simulink model "swingup_control"  (R2021a)
settings: Solver=VariableStepAuto  StartTime=0.0  StopTime=10  RelTol=1e-3
undefined symbols (not defined in the file): A, alpha, B, beta, bm, bp, C, fs_IMU, g, J1, Jw, Ke, Ken, Kt, Ku, Kw, L, La, Ra, real_acc_height, t_noise, V_nom, w_deriv, wacc_LPF, wd_IMU, wgyro_LPF, wn, x0, x0_sw
libraries: spsFirstOrderFilterLib x4, simulink x3, dsparch4 x1, dspsigops x1
settings Model: Creator=jpss8  LastModifiedBy=jpss8

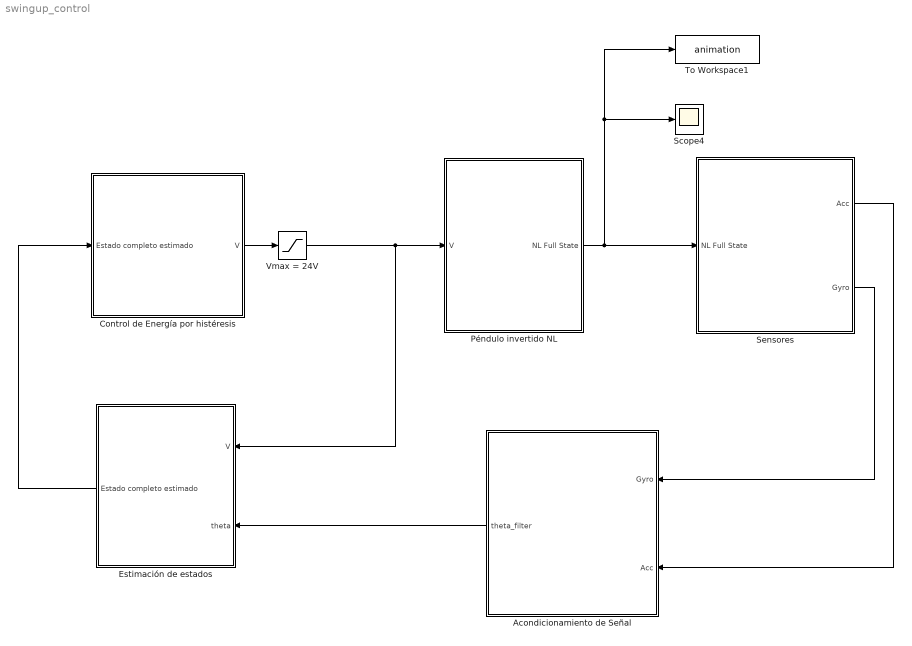
== system swingup_control ==
  Acondicionamiento de Señal : Subsystem
  Control de Energía por histéresis : Subsystem
  Estimación de estados : Subsystem
  Péndulo invertido NL : Subsystem
  Scope4 : Scope
  Sensores : Subsystem
  To Workspace1 : ToWorkspace  VariableName=animation  SaveFormat=Structure With Time  SampleTime=-1
  Vmax = 24V : Saturate  UpperLimit=V_nom  LowerLimit=-V_nom
  wires:
  Vmax = 24V/1 -> Estimación de estados/1(V), Péndulo invertido NL/1(V)
  Sensores/2(Gyro) -> Acondicionamiento de Señal/1(Gyro)
  Acondicionamiento de Señal/1(theta_filter) -> Estimación de estados/2(theta)
  Estimación de estados/1(Estado completo estimado) -> Control de Energía por histéresis/1(Estado completo estimado)
  Sensores/1(Acc) -> Acondicionamiento de Señal/2(Acc)
  Péndulo invertido NL/1(NL Full State) -> To Workspace1/1, Scope4/1, Sensores/1(NL Full State)
  Control de Energía por histéresis/1(V) -> Vmax = 24V/1

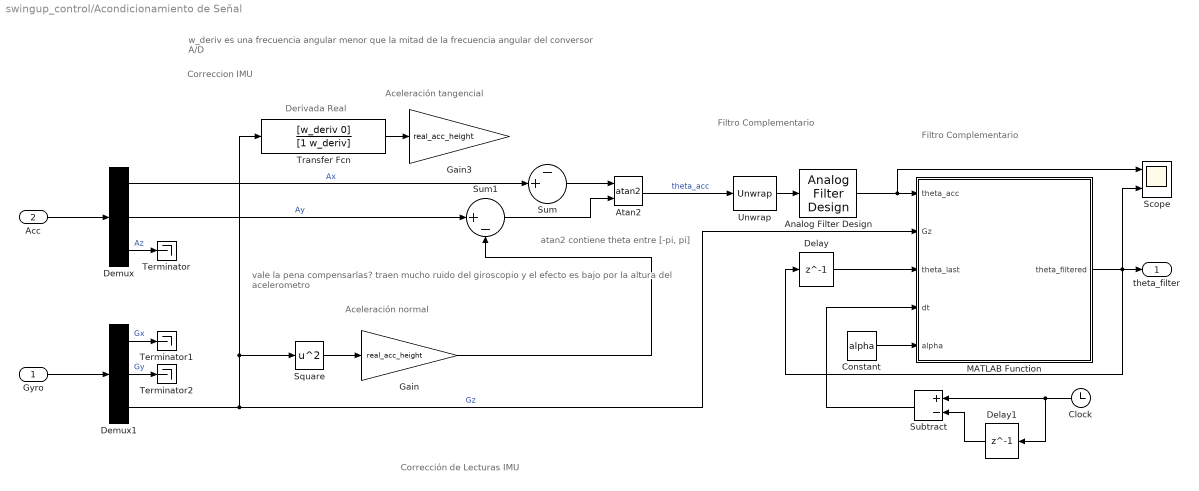
== system swingup_control/Acondicionamiento de Señal ==
  note: vale la pena compensarlas? traen mucho ruido del giroscopio y el efecto es bajo por la altura del acelerometro
  note: w_deriv es una frecuencia angular menor que la mitad de la frecuencia angular del conversor A/D
  note: Derivada Real
  note: atan2 contiene theta entre [-pi, pi]
  note: Correccion IMU
  note: Filtro Complementario
  note: Filtro Complementario
  note: Aceleración tangencial
  note: Aceleración normal
  note: Corrección de Lecturas IMU
  Gyro : Inport
  Acc : Inport  Port=2
  Analog Filter Design : dsparch4/Analog Filter Design  method=Butterworth  filttype=Lowpass  N=1  Wlo=wacc_LPF  Whi=80  Rp=2  Rs=40
  Atan2 : Trigonometry  Operator=atan2
  Clock : Clock
  Constant : Constant  Value=alpha
  Delay : Delay  DelayLength=1  InitialCondition=x0_sw(1)  SampleTime=1/fs_IMU
  Delay1 : Delay  DelayLength=1  InitialCondition=0  SampleTime=1/fs_IMU
  Demux : Demux  Outputs=3
  Demux1 : Demux  Outputs=3
  Gain : Gain  Gain=real_acc_height
  Gain3 : Gain  Gain=real_acc_height
  MATLAB Function : MATLAB Function  TreatAsAtomicUnit=on
  Scope : Scope  NumInputPorts=2
  Square : Math  Operator=square  SaturateOnIntegerOverflow=on
  Subtract : Sum  Inputs=+-
  Sum : Sum  Inputs=-+|
  Sum1 : Sum  Inputs=|+-
  Terminator : Terminator
  Terminator1 : Terminator
  Terminator2 : Terminator
  Transfer Fcn : TransferFcn  Numerator=[w_deriv 0]  Denominator=[1 w_deriv]
  Unwrap : dspsigops/Unwrap  tol=pi  InputProcessing=Columns as channels (frame based)  running=off
  theta_filter : Outport
  wires:
  Gyro/1 -> Demux1/1
  Acc/1 -> Demux/1
  Demux/1 -> Sum/2  "Ax"
  Demux/3 -> Terminator/1  "Az"
  Demux1/1 -> Terminator1/1  "Gx"
  Demux1/2 -> Terminator2/1  "Gy"
  Demux1/3 -> MATLAB Function/2(Gz), Square/1, Transfer Fcn/1  "Gz"
  MATLAB Function/1(theta_filtered) -> Scope/2, theta_filter/1, Delay/1
  Delay/1 -> MATLAB Function/3(theta_last)
  Atan2/1 -> Unwrap/1  "theta_acc"
  Demux/2 -> Sum1/1  "Ay"
  Sum1/1 -> Atan2/2
  Square/1 -> Gain/1
  Sum/1 -> Atan2/1
  Clock/1 -> Subtract/1, Delay1/1
  Delay1/1 -> Subtract/2
  Subtract/1 -> MATLAB Function/4(dt)
  Constant/1 -> MATLAB Function/5(alpha)
  Unwrap/1 -> Analog Filter Design/1
  Analog Filter Design/1 -> Scope/1, MATLAB Function/1(theta_acc)
  Transfer Fcn/1 -> Gain3/1
  Gain/1 -> Sum1/2

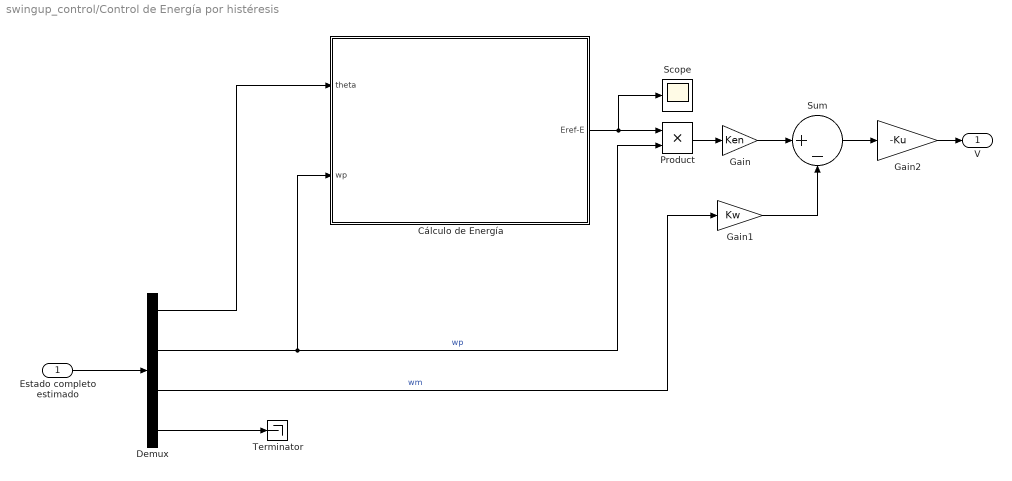
== system swingup_control/Control de Energía por histéresis ==
  Estado completo estimado : Inport
  Cálculo de Energía : Subsystem
  Demux : Demux
  Gain : Gain  Gain=Ken
  Gain1 : Gain  Gain=Kw
  Gain2 : Gain  Gain=-Ku
  Product : Product
  Scope : Scope
  Sum : Sum  Inputs=|+-
  Terminator : Terminator
  V : Outport
  wires:
  Cálculo de Energía/1(Eref-E) -> Scope/1, Product/1
  Estado completo estimado/1 -> Demux/1
  Demux/2 -> Product/2, Cálculo de Energía/2(wp)  "wp"
  Product/1 -> Gain/1
  Gain/1 -> Sum/1
  Demux/3 -> Gain1/1  "wm"
  Gain1/1 -> Sum/2
  Sum/1 -> Gain2/1
  Demux/4 -> Terminator/1
  Demux/1 -> Cálculo de Energía/1(theta)
  Gain2/1 -> V/1

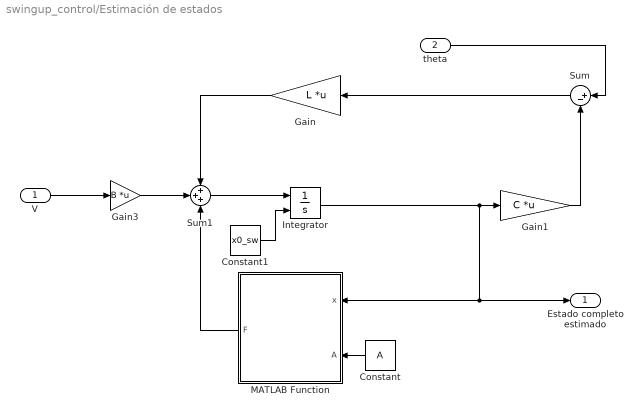
== system swingup_control/Estimación de estados ==
  V : Inport
  theta : Inport  Port=2
  Constant : Constant  Value=A
  Constant1 : Constant  Value=x0_sw
  Gain : Gain  Gain=L  Multiplication=Matrix(K*u)
  Gain1 : Gain  Gain=C  Multiplication=Matrix(K*u)
  Gain3 : Gain  Gain=B  Multiplication=Matrix(K*u)
  Integrator : Integrator  InitialConditionSource=external  InitialCondition=x0
  MATLAB Function : MATLAB Function  TreatAsAtomicUnit=on
  Sum : Sum  Inputs=|+-
  Sum1 : Sum  Inputs=+++
  Estado completo estimado : Outport
  wires:
  theta/1 -> Sum/1
  V/1 -> Gain3/1
  Gain3/1 -> Sum1/2
  Sum1/1 -> Integrator/1
  MATLAB Function/1(F) -> Sum1/3
  Sum/1 -> Gain/1
  Gain1/1 -> Sum/2
  Gain/1 -> Sum1/1
  Constant/1 -> MATLAB Function/2(A)
  Constant1/1 -> Integrator/2
  Integrator/1 -> Estado completo estimado/1, MATLAB Function/1(x), Gain1/1

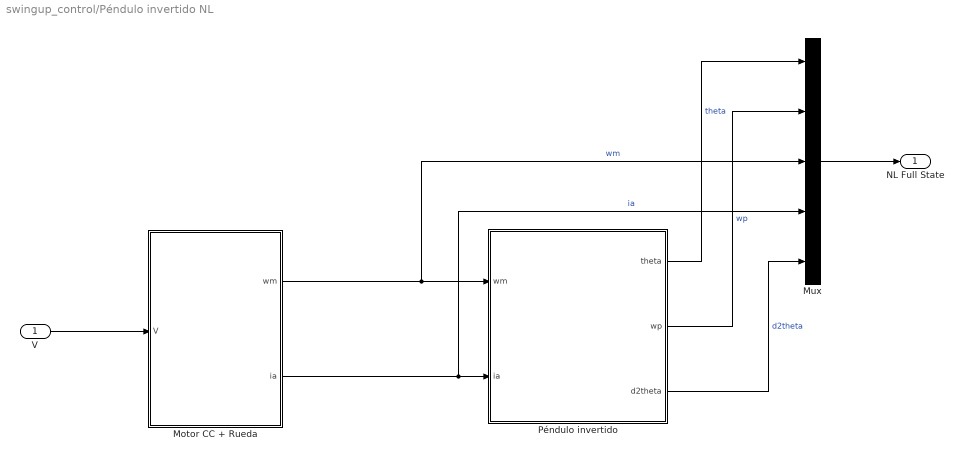
== system swingup_control/Péndulo invertido NL ==
  V : Inport
  Motor CC + Rueda : Subsystem
  Mux : Mux  Inputs=5
  Péndulo invertido : Subsystem
  NL Full State : Outport
  wires:
  Mux/1 -> NL Full State/1
  Péndulo invertido/2(wp) -> Mux/2  "wp"
  Péndulo invertido/1(theta) -> Mux/1  "theta"
  Motor CC + Rueda/1(wm) -> Mux/3, Péndulo invertido/1(wm)  "wm"
  Motor CC + Rueda/2(ia) -> Péndulo invertido/2(ia), Mux/4  "ia"
  V/1 -> Motor CC + Rueda/1(V)
  Péndulo invertido/3(d2theta) -> Mux/5  "d2theta"

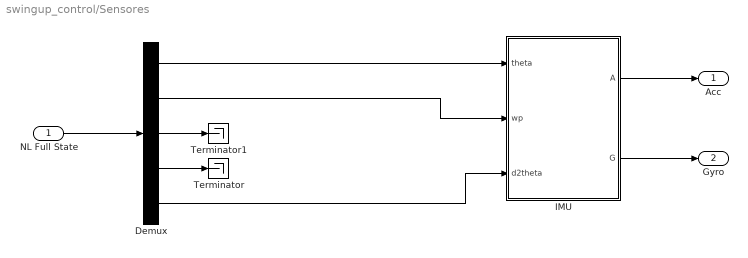
== system swingup_control/Sensores ==
  NL Full State : Inport
  Demux : Demux  Outputs=5
  IMU : Subsystem
  Terminator : Terminator
  Terminator1 : Terminator
  Acc : Outport
  Gyro : Outport  Port=2
  wires:
  NL Full State/1 -> Demux/1
  Demux/2 -> IMU/2(wp)
  Demux/1 -> IMU/1(theta)
  Demux/4 -> Terminator/1
  IMU/2(G) -> Gyro/1
  IMU/1(A) -> Acc/1
  Demux/5 -> IMU/3(d2theta)
  Demux/3 -> Terminator1/1

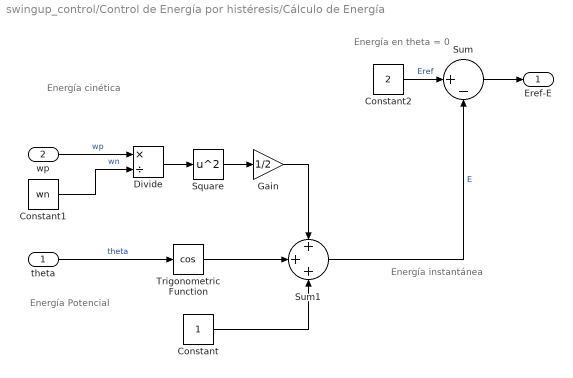
== system swingup_control/Control de Energía por histéresis/Cálculo de Energía ==
  note: Energía Potencial
  note: Energía cinética
  note: Energía instantánea
  note: Energía en theta = 0
  theta : Inport
  wp : Inport  Port=2
  Constant : Constant
  Constant1 : Constant  Value=wn
  Constant2 : Constant  Value=2
  Divide : Product  Inputs=*/
  Gain : Gain  Gain=1/2
  Square : Math  Operator=square  SaturateOnIntegerOverflow=on
  Sum : Sum  Inputs=|+-
  Sum1 : Sum  Inputs=+++
  Trigonometric Function : Trigonometry  Operator=cos
  Eref-E : Outport
  wires:
  Sum/1 -> Eref-E/1
  Constant2/1 -> Sum/1  "Eref"
  Sum1/1 -> Sum/2  "E"
  Constant/1 -> Sum1/3
  Trigonometric Function/1 -> Sum1/2
  theta/1 -> Trigonometric Function/1  "theta"
  Divide/1 -> Square/1
  wp/1 -> Divide/1  "wp"
  Constant1/1 -> Divide/2  "wn"
  Square/1 -> Gain/1
  Gain/1 -> Sum1/1

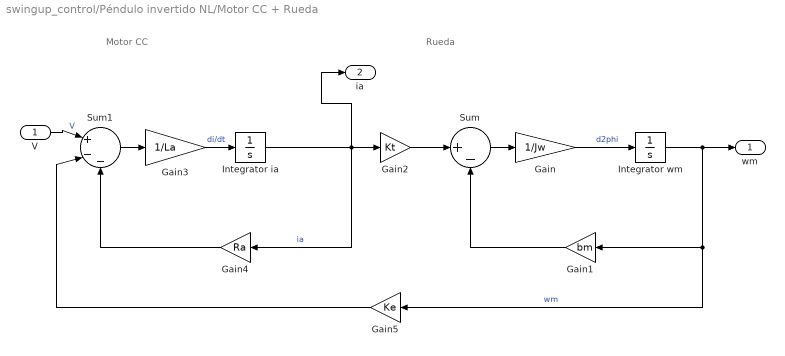
== system swingup_control/Péndulo invertido NL/Motor CC + Rueda ==
  note: Rueda
  note: Motor CC
  V : Inport
  Gain : Gain  Gain=1/Jw
  Gain1 : Gain  Gain=bm
  Gain2 : Gain  Gain=Kt
  Gain3 : Gain  Gain=1/La
  Gain4 : Gain  Gain=Ra
  Gain5 : Gain  Gain=Ke
  Integrator ia : Integrator  InitialCondition=x0_sw(4)
  Integrator wm : Integrator  InitialCondition=x0_sw(3)
  Sum : Sum  Inputs=|+-
  Sum1 : Sum  Inputs=|+--
  wm : Outport
  ia : Outport  Port=2
  wires:
  Sum/1 -> Gain/1
  Gain/1 -> Integrator wm/1  "d2phi"
  Integrator wm/1 -> wm/1, Gain1/1, Gain5/1  "wm"
  Gain1/1 -> Sum/2
  Gain3/1 -> Integrator ia/1  "di/dt"
  Sum1/1 -> Gain3/1
  Gain4/1 -> Sum1/3
  V/1 -> Sum1/1  "V"
  Gain5/1 -> Sum1/2
  Integrator ia/1 -> Gain4/1, ia/1, Gain2/1  "ia"
  Gain2/1 -> Sum/1

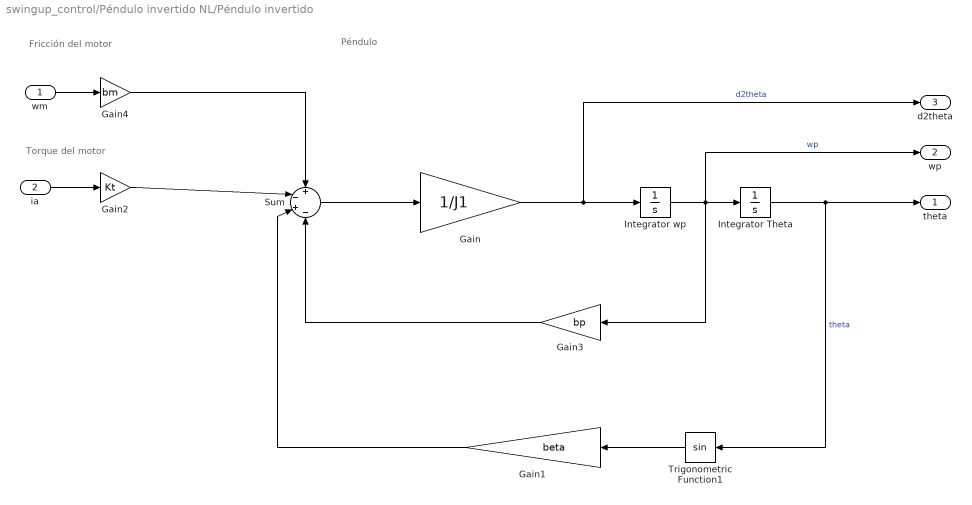
== system swingup_control/Péndulo invertido NL/Péndulo invertido ==
  note: Péndulo
  note: Fricción del motor
  note: Torque del motor
  wm : Inport
  ia : Inport  Port=2
  Gain : Gain  Gain=1/J1
  Gain1 : Gain  Gain=beta
  Gain2 : Gain  Gain=Kt
  Gain3 : Gain  Gain=bp
  Gain4 : Gain  Gain=bm
  Integrator Theta : Integrator  InitialCondition=x0_sw(1)  WrappedStateUpperValue=2*pi  WrappedStateLowerValue=0
  Integrator wp : Integrator  InitialCondition=x0_sw(2)
  Sum : Sum  Inputs=+-+-
  Trigonometric Function1 : Trigonometry
  theta : Outport
  wp : Outport  Port=2
  d2theta : Outport  Port=3
  wires:
  Trigonometric Function1/1 -> Gain1/1
  Gain/1 -> d2theta/1, Integrator wp/1  "d2theta"
  Sum/1 -> Gain/1
  Integrator Theta/1 -> Trigonometric Function1/1, theta/1  "theta"
  Integrator wp/1 -> wp/1, Gain3/1, Integrator Theta/1  "wp"
  Gain3/1 -> Sum/4
  Gain1/1 -> Sum/3
  ia/1 -> Gain2/1
  Gain2/1 -> Sum/2
  wm/1 -> Gain4/1
  Gain4/1 -> Sum/1

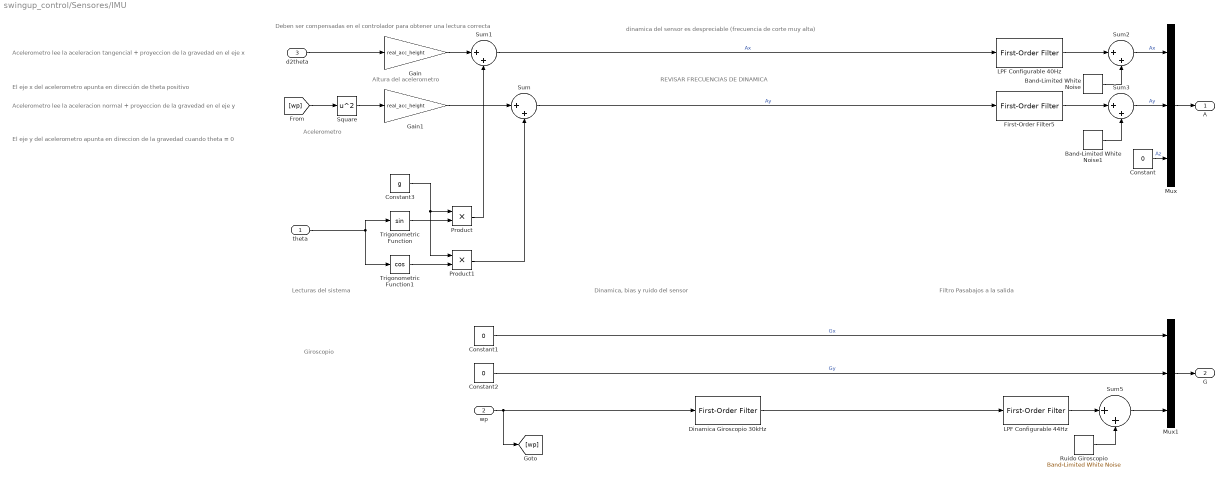
== system swingup_control/Sensores/IMU ==
  note: REVISAR FRECUENCIAS DE DINAMICA
  note: dinamica del sensor es despreciable (frecuencia de corte muy alta)
  note: Dinamica, bias y ruido del sensor
  note: Lecturas del sistema
  note: Acelerometro
  note: Deben ser compensadas en el controlador para obtener una lectura correcta
  note: Acelerometro lee la aceleracion tangencial + proyeccion de la gravedad en el eje x
  note: Altura del acelerometro
  note: El eje y del acelerometro apunta en direccion de la gravedad cuando theta = 0
  note: El eje x del acelerometro apunta en dirección de theta positivo
  note: Acelerometro lee la aceleracion normal + proyeccion de la gravedad en el eje y
  note: Giroscopio
  note: Filtro Pasabajos a la salida
  theta : Inport
  wp : Inport  Port=2
  d2theta : Inport  Port=3
  Band-Limited White Noise : simulink/Sources/Band-Limited White Noise  Cov=acc_noise_power  Ts=t_noise  seed=[23341]
  Band-Limited White Noise1 : simulink/Sources/Band-Limited White Noise  Cov=acc_noise_power  Ts=t_noise  seed=[23341]
  Constant : Constant  Value=0
  Constant1 : Constant  Value=0
  Constant2 : Constant  Value=0
  Constant3 : Constant  Value=g
  Dinamica Giroscopio 30kHz : spsFirstOrderFilterLib/First-Order Filter  FilterType=Lowpass  Tc=2*pi/wd_IMU  Ts=0  Initialize=on  Vac_Init=[0, 0, 60]  Vdc_Init=0  PlotResponse=off  FreqRange="[0,  200,  1]"
  First-Order Filter5 : spsFirstOrderFilterLib/First-Order Filter  FilterType=Lowpass  Tc=2*pi/wacc_LPF  Ts=0  Initialize=on  Vac_Init=[0, 0, 60]  Vdc_Init=0  PlotResponse=off  FreqRange="[0,  200,  1]"
  Gain : Gain  Gain=real_acc_height
  Gain1 : Gain  Gain=real_acc_height
  LPF Configurable 40Hz : spsFirstOrderFilterLib/First-Order Filter  FilterType=Lowpass  Tc=2*pi/wacc_LPF  Ts=0  Initialize=on  Vac_Init=[0, 0, 60]  Vdc_Init=0  PlotResponse=off  FreqRange="[0,  200,  1]"
  LPF Configurable 44Hz : spsFirstOrderFilterLib/First-Order Filter  FilterType=Lowpass  Tc=2*pi/wgyro_LPF  Ts=0  Initialize=on  Vac_Init=[0, 0, 60]  Vdc_Init=0  PlotResponse=off  FreqRange="[0,  200,  1]"
  Mux : Mux  Inputs=3
  Mux1 : Mux  Inputs=3
  Product : Product
  Product1 : Product
  Ruido Giroscopio : simulink/Sources/Band-Limited White Noise  Cov=gyro_noise_power  Ts=t_noise  seed=[23341]
  Square : Math  Operator=square  SaturateOnIntegerOverflow=on
  Sum{,1..3,5} (5 alike) : Sum  Inputs=|++
  Trigonometric Function : Trigonometry
  Trigonometric Function1 : Trigonometry  Operator=cos
  A : Outport
  G : Outport  Port=2
  wires:
  Constant2/1 -> Mux1/2  "Gy"
  Constant1/1 -> Mux1/1  "Gx"
  Trigonometric Function/1 -> Product/2
  Trigonometric Function1/1 -> Product1/2
  Constant3/1 -> Product1/1, Product/1
  Product1/1 -> Sum/2
  Product/1 -> Sum1/2
  Gain1/1 -> Sum/1
  theta/1 -> Trigonometric Function1/1, Trigonometric Function/1
  Gain/1 -> Sum1/1
  d2theta/1 -> Gain/1
  Square/1 -> Gain1/1
  Constant/1 -> Mux/3  "Az"
  Sum1/1 -> LPF Configurable 40Hz/1  "Ax"
  Band-Limited White Noise/1 -> Sum2/2
  Band-Limited White Noise1/1 -> Sum3/2
  Ruido Giroscopio/1 -> Sum5/2
  Dinamica Giroscopio 30kHz/1 -> LPF Configurable 44Hz/1
  wp/1 -> Dinamica Giroscopio 30kHz/1, [wp]
  Mux/1 -> A/1
  Mux1/1 -> G/1
  Sum2/1 -> Mux/1  "Ax"
  Sum3/1 -> Mux/2  "Ay"
  [wp] -> Square/1
  Sum/1 -> First-Order Filter5/1  "Ay"
  Sum5/1 -> Mux1/3
  First-Order Filter5/1 -> Sum3/1
  LPF Configurable 40Hz/1 -> Sum2/1
  LPF Configurable 44Hz/1 -> Sum5/1

== matlab function swingup_control/Estimación de estados/MATLAB Function ==
  data: x input; F output; A input
function F = CampoVectorial(x, A)

k = A(2,1);
A(2,1) = 0;

F = A*x;
F(2) = F(2) + k * sin(x(1));

== matlab function swingup_control/Acondicionamiento de Señal/MATLAB Function ==
  data: theta_acc input; theta_filtered output; Gz input; theta_last input; dt input; alpha input
function theta_filtered = complementaryFilter(theta_acc, Gz, theta_last, dt, alpha)
theta_gy = Gz * dt;
theta_filtered = theta_acc*(1-alpha) + alpha * (theta_last + theta_gy);
end
